simulink model "DFIG"  (Simulink 7.8)
settings: Solver=ode45  StartTime=0.0  StopTime=10.0  RelTol=1e-3
values from neighbouring files (symbols this model uses):
  ps_simStepTime = 5e-6    (= 5e-06)    [plotSimOutput.m]
undefined symbols (not defined in the file or in its folder): D1, Delta, flt_fin_time, flt_start_time, pm_enable_fault, pm_enable_swell, pm_f, pm_fault_type, pm_faultL_H, pm_faultLength, pm_faultR_Ohm, pm_faultStart, pm_gridL_H, pm_gridR_Ohm, pm_initial_angle, pm_multiFault1_end, pm_multiFault1_start, pm_multiFault1L_H, pm_multiFault1R_Ohm, pm_multiFault2_end, pm_multiFault2_start, pm_multiFault2L_H, pm_multiFault2R_Ohm, pm_multiFault3_end, pm_multiFault3_start, pm_multiFault3L_H, pm_multiFault3R_Ohm, pm_multiFault4_end, pm_multiFault4_start, pm_multiFault4L_H, pm_multiFault4R_Ohm, pm_swellaangle_1, pm_swellaangle_2, pm_swellaangle_3, pm_swellbangle_1, pm_swellbangle_2, pm_swellbangle_3, pm_swellcangle_1, pm_swellcangle_2, pm_swellcangle_3, pm_swellEnd, pm_swellPh1_1, pm_swellPh1_2, pm_swellPh1_3, pm_swellPh2_1, pm_swellPh2_2, pm_swellPh2_3, pm_swellPh3_1, pm_swellPh3_2, pm_swellPh3_3, pm_swellStart1, pm_swellStart2, pm_swellStart3, pm_Vg_pp, pm_WTtrafo_L_pu, pm_WTtrafo_Pn_VA, pm_WTtrafo_R_pu, pm_WTtrafo_V2phph_Vrms
libraries: powerlib x39, simulink x4
settings Model: Creator=CNFELUO1  LastModifiedBy=CNFELUO1

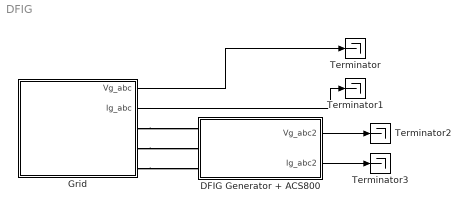
== system DFIG ==
  DFIG Generator + ACS800 : Subsystem
  Grid : Subsystem
  Terminator{,1..3} (4 alike) : Terminator
  wires:
  Grid/1(Vg_abc) -> Terminator/1
  Grid/2(Ig_abc) -> Terminator1/1
  DFIG Generator + ACS800/1(Vg_abc2) -> Terminator2/1
  DFIG Generator + ACS800/2(Ig_abc2) -> Terminator3/1
  connections:
  Grid/RConn3 -- DFIG Generator + ACS800/LConn3
  Grid/RConn2 -- DFIG Generator + ACS800/LConn2
  Grid/RConn1 -- DFIG Generator + ACS800/LConn1

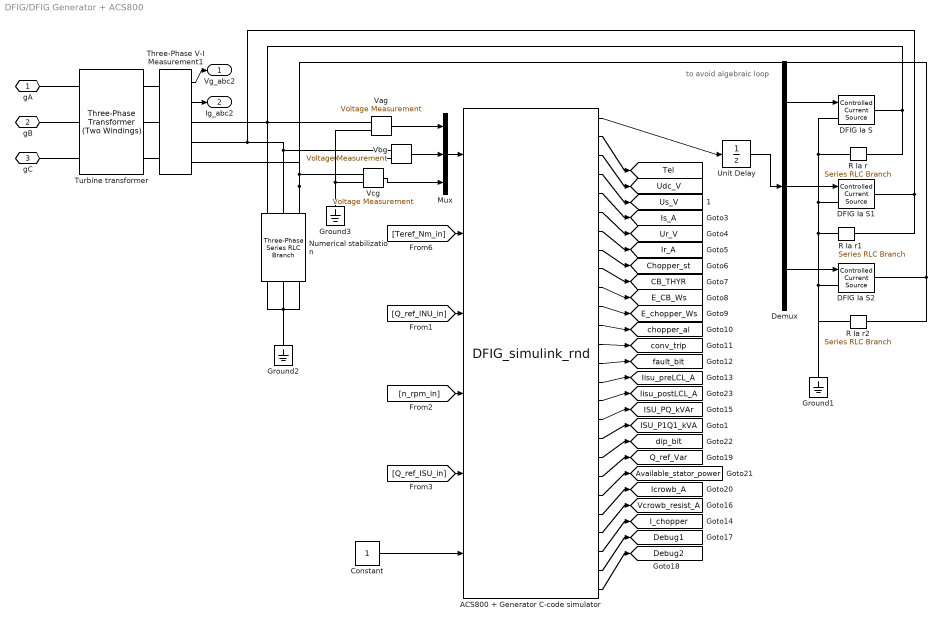
== system DFIG/DFIG Generator + ACS800 ==
  note: to avoid algebraic loop
  ACS800 + Generator C-code simulator : S-Function  FunctionName=DFIG_simulink_rnd  EnableBusSupport=off
      mask Display:
      | port_label('output',1,'Ig_A')
      | port_label('output',2,'Tel')
      | port_label('output',3,'Udc_V')
      | port_label('output',4,'Us_V')
      | port_label('output',5,'Is_A')
      | port_label('output',6,'Ur_V')
      | port_label('output',7,'Ir_A')
      | port_label('output',8,'chopper_st')
      | port_label('output',9,'CB_THYR')
      | port_label('output',10,'E_CB_Ws')
      | port_label('output',11,'E_chopper_Ws')
      | port_label('output',12,'chopper_al')
      | port_label('output',13,'conv_trip')
      | port_label('output',14,'fault_bit')
      | port_label('output',15,'Iisu_preLCL_A')
      | port_label('output',16,'Iisu_postLCL_A')
      | port_label('output',17,'ISU_PQ_kVA')
      | port_label('output',18,'ISU_P1Q1_kVA')
      | port_label('output',19,'dip_bit')
      | port_label('output',20,'Q_ref_VAr')
      | port_label('output',21,'Stator P lim')
      | port_label('output',22,'Icrowb_A')
      | port_label('output',23,'Vcrowb_resist_A')
      | port_label('output',24,'I_chopper')
      | port_label('output',25,'Debug1')
      | port_label('output',26,'Debug2')
      | 
      | port_label('input',1,'Vg_V')
      | port_label('input',2,'Teref_Nm_in')
      | port_label('input',3,'Q_ref_INU_in')
      | port_label('input',4,'n_rpm_in')
      | port_label('input',5,'Q_ref_ISU_in')
      | port_label('input',6,'Enable')
  Constant : Constant
  DFIG Ia S : powerlib/Electrical Sources/Controlled Current Source  Initialize=off  Source_Type=AC  Amplitude=0  Phase=0  Frequency=0  Measurements=None
  DFIG Ia S1 : powerlib/Electrical Sources/Controlled Current Source  Initialize=off  Source_Type=AC  Amplitude=0  Phase=0  Frequency=0  Measurements=None
  DFIG Ia S2 : powerlib/Electrical Sources/Controlled Current Source  Initialize=off  Source_Type=AC  Amplitude=0  Phase=0  Frequency=0  Measurements=None
  Demux : Demux  Outputs=3
  Ground1 : powerlib/Elements/Ground  LConnTagsString=a
  Ground2 : powerlib/Elements/Ground  LConnTagsString=a
  Ground3 : powerlib/Elements/Ground  LConnTagsString=a
  Mux : Mux  Inputs=3
  Numerical stabilization : powerlib/Elements/Three-Phase Series RLC Branch  LConnTagsString=A|B|C  RConnTagsString=A|B|C  BranchType=RC  Resistance=1  Inductance=1e-3  Capacitance=30e-6  Measurements=None
  R Ia r : powerlib/Elements/Series RLC Branch  LConnTagsString=__new0  RConnTagsString=__new0  BranchType=R  Resistance=10e6  Inductance=1e-3  SetiL0=off  InitialCurrent=0  Capacitance=1e-6  Setx0=off  InitialVoltage=0  Measurements=None
  R Ia r1 : powerlib/Elements/Series RLC Branch  LConnTagsString=__new0  RConnTagsString=__new0  BranchType=R  Resistance=10e6  Inductance=1e-3  SetiL0=off  InitialCurrent=0  Capacitance=1e-6  Setx0=off  InitialVoltage=0  Measurements=None
  R Ia r2 : powerlib/Elements/Series RLC Branch  LConnTagsString=__new0  RConnTagsString=__new0  BranchType=R  Resistance=10e6  Inductance=1e-3  SetiL0=off  InitialCurrent=0  Capacitance=1e-6  Setx0=off  InitialVoltage=0  Measurements=None
  Three-Phase V-I Measurement1 : powerlib/Measurements/Three-Phase V-I Measurement  VoltageMeasurement=phase-to-ground  SetLabelV=off  LabelV=Vabc  Vpu=off  VpuLL=off  CurrentMeasurement=yes  SetLabelI=off  LabelI=Iabc  Ipu=off  Pbase=100e6  Vbase=500e3  OutputType=Complex  PhasorSimulation=off  PSBequivalent=0
  Turbine transformer : powerlib/Elements/Three-Phase Transformer (Two Windings)  Winding1Connection=Delta (D1)  UNITS=pu  NominalPower=[ pm_WTtrafo_Pn_VA , pm_f ]  Winding1=[pm_Vg_pp , 0.5*pm_WTtrafo_R_pu , 0.5*pm_WTtrafo_L_pu ]  Winding2Connection=Yg  Winding2=[pm_WTtrafo_V2phph_Vrms , 0.5*pm_WTtrafo_R_pu , 0.5*pm_WTtrafo_L_pu ]  SetSaturation=off  Rm=500  Lm=500  Saturation=[ 0,0 ; 0.0024,1.2 ; 1.0,1.52 ]  Hysteresis=off  DataFile='hysteresis'  SetInitialFlux=off  InitialFluxes=[ 0.8 , -0.8 , 0.7 ]  Measurements=None  MoreParameters=off  BreakLoop=off  DataType=off  TransfoNumber=1
  Unit Delay : UnitDelay  SampleTime=-1
  Vag : powerlib/Measurements/Voltage Measurement  PhasorSimulation=off  OutputType=Complex  PSBequivalent=0
  Vbg : powerlib/Measurements/Voltage Measurement  PhasorSimulation=off  OutputType=Complex  PSBequivalent=0
  Vcg : powerlib/Measurements/Voltage Measurement  PhasorSimulation=off  OutputType=Complex  PSBequivalent=0
  gA : PMIOPort  Port=1  Side=Left
  gB : PMIOPort  Port=2  Side=Left
  gC : PMIOPort  Port=3  Side=Left
  Vg_abc2 : Outport
  Ig_abc2 : Outport  Port=2
  tag scope: Available_stator_power=global, CB_THYR=global, Chopper_st=global, Debug1=global, Debug2=global, E_CB_Ws=global, E_chopper_Ws=global, ISU_P1Q1_kVA=global, ISU_PQ_kVAr=global, I_chopper=global, Icrowb_A=global, Iisu_postLCL_A=global, Iisu_preLCL_A=global, Ir_A=global, Is_A=global, Q_ref_Var=global, Tel=global, Udc_V=global, Ur_V=global, Us_V=global, Vcrowb_resist_A=global, chopper_al=global, conv_trip=global, dip_bit=global, fault_bit=global
  wires:
  ACS800 + Generator C-code simulator/15 -> [Iisu_preLCL_A]
  ACS800 + Generator C-code simulator/14 -> [fault_bit]
  ACS800 + Generator C-code simulator/13 -> [conv_trip]
  ACS800 + Generator C-code simulator/12 -> [chopper_al]
  ACS800 + Generator C-code simulator/11 -> [E_chopper_Ws]
  ACS800 + Generator C-code simulator/10 -> [E_CB_Ws]
  ACS800 + Generator C-code simulator/9 -> [CB_THYR]
  ACS800 + Generator C-code simulator/8 -> [Chopper_st]
  ACS800 + Generator C-code simulator/7 -> [Ir_A]
  ACS800 + Generator C-code simulator/6 -> [Ur_V]
  ACS800 + Generator C-code simulator/5 -> [Is_A]
  ACS800 + Generator C-code simulator/4 -> [Us_V]
  ACS800 + Generator C-code simulator/3 -> [Udc_V]
  ACS800 + Generator C-code simulator/2 -> [Tel]
  Demux/1 -> DFIG Ia S/1
  ACS800 + Generator C-code simulator/1 -> Unit Delay/1
  Mux/1 -> ACS800 + Generator C-code simulator/1
  Demux/2 -> DFIG Ia S1/1
  Demux/3 -> DFIG Ia S2/1
  Unit Delay/1 -> Demux/1
  [Teref_Nm_in] -> ACS800 + Generator C-code simulator/2
  [Q_ref_INU_in] -> ACS800 + Generator C-code simulator/3
  [n_rpm_in] -> ACS800 + Generator C-code simulator/4
  [Q_ref_ISU_in] -> ACS800 + Generator C-code simulator/5
  Vcg/1 -> Mux/3
  Vbg/1 -> Mux/2
  Vag/1 -> Mux/1
  Constant/1 -> ACS800 + Generator C-code simulator/6
  ACS800 + Generator C-code simulator/16 -> [Iisu_postLCL_A]
  ACS800 + Generator C-code simulator/17 -> [ISU_PQ_kVAr]
  ACS800 + Generator C-code simulator/18 -> [ISU_P1Q1_kVA]
  ACS800 + Generator C-code simulator/19 -> [dip_bit]
  ACS800 + Generator C-code simulator/20 -> [Q_ref_Var]
  ACS800 + Generator C-code simulator/21 -> [Available_stator_power]
  ACS800 + Generator C-code simulator/22 -> [Icrowb_A]
  ACS800 + Generator C-code simulator/23 -> [Vcrowb_resist_A]
  ACS800 + Generator C-code simulator/24 -> [I_chopper]
  ACS800 + Generator C-code simulator/25 -> [Debug1]
  ACS800 + Generator C-code simulator/26 -> [Debug2]
  Three-Phase V-I Measurement1/1 -> Vg_abc2/1
  Three-Phase V-I Measurement1/2 -> Ig_abc2/1
  connections:
  Vag/LConn1 -- R Ia r/RConn1 -- DFIG Ia S/RConn1 -- Numerical stabilization/LConn1 -- Three-Phase V-I Measurement1/RConn1
  DFIG Ia S2/RConn1 -- R Ia r2/RConn1 -- Numerical stabilization/LConn3 -- Vcg/LConn1 -- Three-Phase V-I Measurement1/RConn3
  R Ia r1/LConn1 -- R Ia r2/LConn1 -- Ground1/LConn1 -- DFIG Ia S2/LConn1 -- DFIG Ia S1/LConn1 -- DFIG Ia S/LConn1 -- R Ia r/LConn1
  Ground2/LConn1 -- Numerical stabilization/RConn2 -- Numerical stabilization/RConn3 -- Numerical stabilization/RConn1
  Vag/LConn2 -- Vbg/LConn2 -- Ground3/LConn1 -- Vcg/LConn2
  gC/RConn1 -- Turbine transformer/LConn3
  gB/RConn1 -- Turbine transformer/LConn2
  gA/RConn1 -- Turbine transformer/LConn1
  Turbine transformer/RConn1 -- Three-Phase V-I Measurement1/LConn1
  Turbine transformer/RConn2 -- Three-Phase V-I Measurement1/LConn2
  Turbine transformer/RConn3 -- Three-Phase V-I Measurement1/LConn3
  Numerical stabilization/LConn2 -- Vbg/LConn1 -- Three-Phase V-I Measurement1/RConn2 -- R Ia r1/RConn1 -- DFIG Ia S1/RConn1

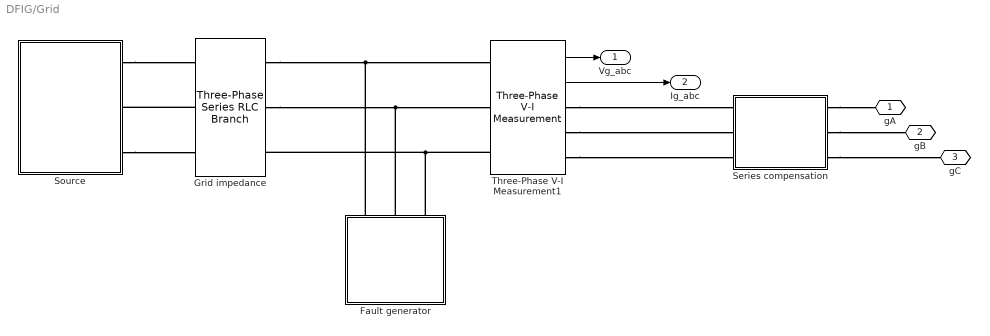
== system DFIG/Grid ==
  Fault generator : Subsystem
  Grid impedance : powerlib/Elements/Three-Phase Series RLC Branch  LConnTagsString=A|B|C  RConnTagsString=A|B|C  BranchType=RL  Resistance=pm_gridR_Ohm  Inductance=pm_gridL_H  Capacitance=[]  Measurements=None
  Series compensation : Subsystem  mask{t_on=3, c=5e-4}
      mask prompts: t_on "Compensation switch on time (s)"; c "Series capacitance (F)"
  Source : Subsystem
  Three-Phase V-I Measurement1 : powerlib/Measurements/Three-Phase V-I Measurement  VoltageMeasurement=phase-to-ground  SetLabelV=off  LabelV=Vabc  Vpu=off  VpuLL=off  CurrentMeasurement=yes  SetLabelI=off  LabelI=Iabc  Ipu=off  Pbase=100e6  Vbase=500e3  OutputType=Complex  PhasorSimulation=off  PSBequivalent=0
  gA : PMIOPort  Port=1  Side=Right
  gB : PMIOPort  Port=2  Side=Right
  gC : PMIOPort  Port=3  Side=Right
  Vg_abc : Outport
  Ig_abc : Outport  Port=2
  wires:
  Three-Phase V-I Measurement1/2 -> Ig_abc/1
  Three-Phase V-I Measurement1/1 -> Vg_abc/1
  connections:
  Three-Phase V-I Measurement1/LConn3 -- Grid impedance/RConn3 -- Fault generator/RConn3
  Grid impedance/RConn2 -- Three-Phase V-I Measurement1/LConn2 -- Fault generator/RConn2
  Grid impedance/RConn1 -- Three-Phase V-I Measurement1/LConn1 -- Fault generator/RConn1
  Source/RConn1 -- Grid impedance/LConn1
  Grid impedance/LConn2 -- Source/RConn2
  Source/RConn3 -- Grid impedance/LConn3
  Three-Phase V-I Measurement1/RConn1 -- Series compensation/RConn1
  Three-Phase V-I Measurement1/RConn2 -- Series compensation/RConn2
  Three-Phase V-I Measurement1/RConn3 -- Series compensation/RConn3
  Series compensation/LConn1 -- gA/RConn1
  Series compensation/LConn2 -- gB/RConn1
  Series compensation/LConn3 -- gC/RConn1

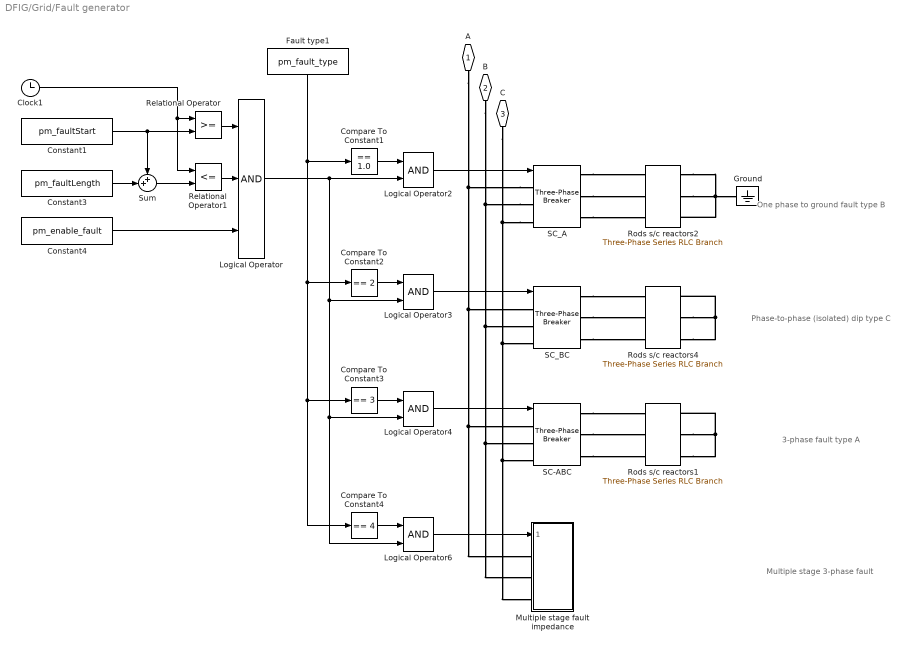
== system DFIG/Grid/Fault generator ==
  note: Multiple stage 3-phase fault
  note: One phase to ground fault
      | type B
  note: 3-phase fault
      | type A
  note: Phase-to-phase (isolated) dip
      | type C
  Clock1 : Clock
  Compare To Constant1 : simulink/Logic and Bit Operations/Compare To Constant  relop===  const=1.0  OutDataTypeStr=uint8
  Compare To Constant2 : simulink/Logic and Bit Operations/Compare To Constant  relop===  const=2  OutDataTypeStr=uint8
  Compare To Constant3 : simulink/Logic and Bit Operations/Compare To Constant  relop===  const=3  OutDataTypeStr=uint8
  Compare To Constant4 : simulink/Logic and Bit Operations/Compare To Constant  relop===  const=4  OutDataTypeStr=uint8
  Constant1 : Constant  Value=pm_faultStart
  Constant3 : Constant  Value=pm_faultLength
  Constant4 : Constant  Value=pm_enable_fault
  Fault type1 : Constant  Value=pm_fault_type
  Ground : powerlib/Elements/Ground  LConnTagsString=a
  Logical Operator : Logic  Inputs=3  AllPortsSameDT=off  OutDataTypeStr=boolean
  Logical Operator{2..4,6} (4 alike) : Logic  AllPortsSameDT=off  OutDataTypeStr=boolean
  Multiple stage fault impedance : Subsystem
  Relational Operator : RelationalOperator  OutDataTypeStr=boolean
  Relational Operator1 : RelationalOperator  Operator=<=  OutDataTypeStr=boolean
  Rods s/c reactors1 : powerlib/Elements/Three-Phase Series RLC Branch  LConnTagsString=A|B|C  RConnTagsString=A|B|C  BranchType=RL  Resistance=pm_faultR_Ohm  Inductance=pm_faultL_H  Capacitance=[]  Measurements=None
  Rods s/c reactors2 : powerlib/Elements/Three-Phase Series RLC Branch  LConnTagsString=A|B|C  RConnTagsString=A|B|C  BranchType=RL  Resistance=pm_faultR_Ohm  Inductance=pm_faultL_H  Capacitance=[]  Measurements=None
  Rods s/c reactors4 : powerlib/Elements/Three-Phase Series RLC Branch  LConnTagsString=A|B|C  RConnTagsString=A|B|C  BranchType=RL  Resistance=pm_faultR_Ohm  Inductance=pm_faultL_H  Capacitance=[]  Measurements=None
  SC-ABC : powerlib/Elements/Three-Phase Breaker  InitialState=open  SwitchA=on  SwitchB=on  SwitchC=on  SwitchTimes="[flt_start_time  flt_fin_time]"  External=on  BreakerResistance=1e-6  SnubberResistance=10000000  SnubberCapacitance=inf  Measurements=None
      settings: AttributesFormatString=\n
  SC_A : powerlib/Elements/Three-Phase Breaker  InitialState=open  SwitchA=on  SwitchB=off  SwitchC=off  SwitchTimes="[flt_start_time  flt_fin_time]"  External=on  BreakerResistance=1e-6  SnubberResistance=10000000  SnubberCapacitance=inf  Measurements=None
      settings: AttributesFormatString=\n
  SC_BC : powerlib/Elements/Three-Phase Breaker  InitialState=open  SwitchA=off  SwitchB=on  SwitchC=on  SwitchTimes="[flt_start_time  flt_fin_time]"  External=on  BreakerResistance=1e-6  SnubberResistance=10000000  SnubberCapacitance=inf  Measurements=None
      settings: AttributesFormatString=\n
  Sum : Sum  Inputs=++|
  A : PMIOPort  Port=1  Side=Right
  B : PMIOPort  Port=2  Side=Right
  C : PMIOPort  Port=3  Side=Right
  wires:
  Clock1/1 -> Relational Operator/1, Relational Operator1/1
  Logical Operator/1 -> Logical Operator6/2, Logical Operator4/2, Logical Operator3/2, Logical Operator2/2
  Constant4/1 -> Logical Operator/3
  Relational Operator1/1 -> Logical Operator/2
  Relational Operator/1 -> Logical Operator/1
  Sum/1 -> Relational Operator1/2
  Constant1/1 -> Relational Operator/2, Sum/1
  Constant3/1 -> Sum/2
  Logical Operator6/1 -> Multiple stage fault impedance/1(Enabled)
  Logical Operator4/1 -> SC-ABC/1
  Logical Operator3/1 -> SC_BC/1
  Logical Operator2/1 -> SC_A/1
  Compare To Constant4/1 -> Logical Operator6/1
  Compare To Constant3/1 -> Logical Operator4/1
  Compare To Constant2/1 -> Logical Operator3/1
  Fault type1/1 -> Compare To Constant4/1, Compare To Constant3/1, Compare To Constant2/1, Compare To Constant1/1
  Compare To Constant1/1 -> Logical Operator2/1
  connections:
  SC_A/LConn1 -- SC_BC/LConn1 -- SC-ABC/LConn1 -- Multiple stage fault impedance/LConn1 -- A/RConn1
  SC_A/LConn2 -- SC_BC/LConn2 -- SC-ABC/LConn2 -- Multiple stage fault impedance/LConn2 -- B/RConn1
  SC_A/LConn3 -- SC_BC/LConn3 -- SC-ABC/LConn3 -- Multiple stage fault impedance/LConn3 -- C/RConn1
  SC_A/RConn1 -- Rods s/c reactors2/LConn1
  SC_A/RConn2 -- Rods s/c reactors2/LConn2
  SC_A/RConn3 -- Rods s/c reactors2/LConn3
  Rods s/c reactors2/RConn2 -- Rods s/c reactors2/RConn3 -- Rods s/c reactors2/RConn1 -- Ground/LConn1
  SC-ABC/RConn1 -- Rods s/c reactors1/LConn1
  SC-ABC/RConn2 -- Rods s/c reactors1/LConn2
  SC-ABC/RConn3 -- Rods s/c reactors1/LConn3
  Rods s/c reactors1/RConn3 -- Rods s/c reactors1/RConn1 -- Rods s/c reactors1/RConn2
  Rods s/c reactors4/RConn2 -- Rods s/c reactors4/RConn1 -- Rods s/c reactors4/RConn3
  SC_BC/RConn1 -- Rods s/c reactors4/LConn1
  SC_BC/RConn2 -- Rods s/c reactors4/LConn2
  SC_BC/RConn3 -- Rods s/c reactors4/LConn3

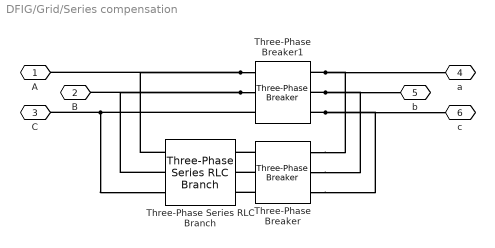
== system DFIG/Grid/Series compensation ==
  Three-Phase Series RLC Branch : powerlib/Elements/Three-Phase Series RLC Branch  LConnTagsString=A|B|C  RConnTagsString=A|B|C  BranchType=C  Resistance=1  Inductance=1e-3  Capacitance=c  Measurements=None
  Three-Phase Breaker : powerlib/Elements/Three-Phase Breaker  InitialState=open  SwitchA=on  SwitchB=on  SwitchC=on  SwitchTimes=[t_on]  External=off  BreakerResistance=0.001  SnubberResistance=1e6  SnubberCapacitance=inf  Measurements=None
  Three-Phase Breaker1 : powerlib/Elements/Three-Phase Breaker  InitialState=closed  SwitchA=on  SwitchB=on  SwitchC=on  SwitchTimes=[t_on]  External=off  BreakerResistance=0.001  SnubberResistance=1e6  SnubberCapacitance=inf  Measurements=None
  A : PMIOPort  Port=1  Side=Right
  B : PMIOPort  Port=2  Side=Right
  C : PMIOPort  Port=3  Side=Right
  a : PMIOPort  Port=4  Side=Left
  b : PMIOPort  Port=5  Side=Left
  c : PMIOPort  Port=6  Side=Left
  connections:
  Three-Phase Breaker1/RConn3 -- c/RConn1 -- Three-Phase Breaker/RConn3
  Three-Phase Breaker1/RConn2 -- b/RConn1 -- Three-Phase Breaker/RConn2
  Three-Phase Breaker1/RConn1 -- a/RConn1 -- Three-Phase Breaker/RConn1
  Three-Phase Breaker/LConn3 -- Three-Phase Series RLC Branch/RConn3
  Three-Phase Breaker/LConn2 -- Three-Phase Series RLC Branch/RConn2
  Three-Phase Breaker/LConn1 -- Three-Phase Series RLC Branch/RConn1
  Three-Phase Breaker1/LConn3 -- C/RConn1 -- Three-Phase Series RLC Branch/LConn3
  Three-Phase Breaker1/LConn2 -- B/RConn1 -- Three-Phase Series RLC Branch/LConn2
  Three-Phase Breaker1/LConn1 -- A/RConn1 -- Three-Phase Series RLC Branch/LConn1

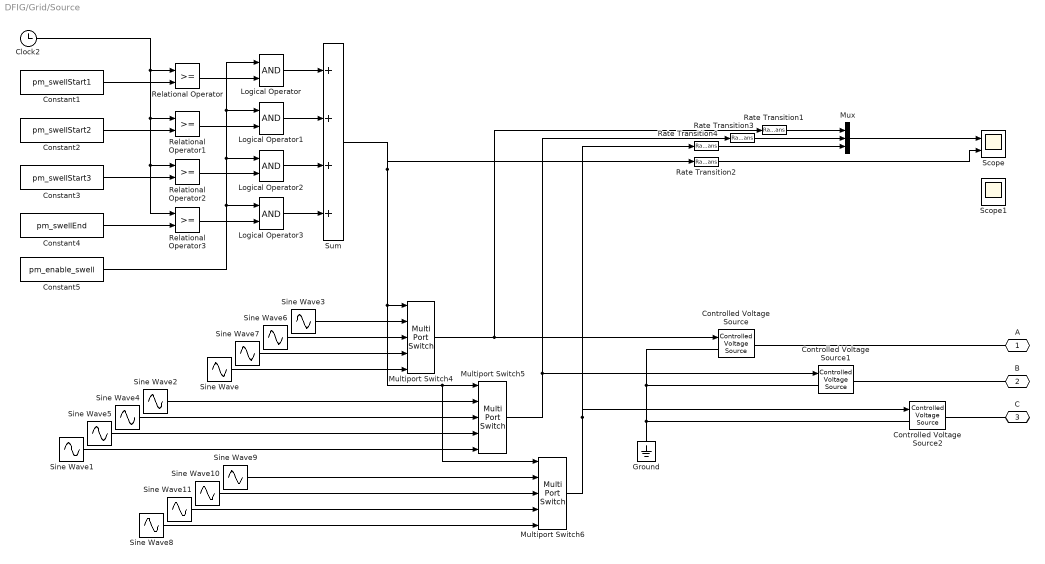
== system DFIG/Grid/Source ==
  Clock2 : Clock
  Constant1 : Constant  Value=pm_swellStart1
  Constant2 : Constant  Value=pm_swellStart2
  Constant3 : Constant  Value=pm_swellStart3
  Constant4 : Constant  Value=pm_swellEnd
  Constant5 : Constant  Value=pm_enable_swell
  Controlled Voltage Source : powerlib/Electrical Sources/Controlled Voltage Source  Initialize=on  Source_Type=AC  Amplitude=0  Phase=0  Frequency=0  Measurements=None
  Controlled Voltage Source1 : powerlib/Electrical Sources/Controlled Voltage Source  Initialize=on  Source_Type=AC  Amplitude=0  Phase=0  Frequency=0  Measurements=None
  Controlled Voltage Source2 : powerlib/Electrical Sources/Controlled Voltage Source  Initialize=on  Source_Type=AC  Amplitude=0  Phase=0  Frequency=0  Measurements=None
  Ground : powerlib/Elements/Ground  LConnTagsString=a
  Logical Operator{,1..3} (4 alike) : Logic  AllPortsSameDT=off  OutDataTypeStr=boolean
  Multiport Switch4 : MultiPortSwitch  Inputs=4  zeroidx=off
  Multiport Switch5 : MultiPortSwitch  Inputs=4  zeroidx=off
  Multiport Switch6 : MultiPortSwitch  Inputs=4  zeroidx=off
  Mux : Mux  Inputs=3
  Rate Transition{1..4} (4 alike) : RateTransition  OutPortSampleTime=500e-6
  Relational Operator{,1..3} (4 alike) : RelationalOperator  OutDataTypeStr=boolean
  Scope : Scope  NumInputPorts=2
      settings: YMin=-30000~-5  YMax=30000~5
  Scope1 : Scope  NumInputPorts=2
      settings: YMin=-30000~-5  YMax=30000~5
  Sine Wave : Sin  Amplitude=pm_Vg_pp*sqrt(2)./sqrt(3)  Frequency=pm_f*2*pi  Phase=pm_initial_angle.*pi./180  SampleTime=ps_simStepTime  VectorParams1D=off
  Sine Wave1 : Sin  Amplitude=pm_Vg_pp*sqrt(2)./sqrt(3)  Frequency=pm_f*2*pi  Phase=pm_initial_angle.*pi./180-2*pi/3  SampleTime=ps_simStepTime  VectorParams1D=off
  Sine Wave10 : Sin  Amplitude=pm_Vg_pp*sqrt(2)./sqrt(3)*pm_swellPh3_2  Frequency=pm_f*2*pi  Phase=pm_initial_angle.*pi./180 + pm_swellcangle_2  SampleTime=ps_simStepTime  VectorParams1D=off
  Sine Wave11 : Sin  Amplitude=pm_Vg_pp*sqrt(2)./sqrt(3)*pm_swellPh3_3  Frequency=pm_f*2*pi  Phase=pm_initial_angle.*pi./180+pm_swellcangle_3  SampleTime=ps_simStepTime  VectorParams1D=off
  Sine Wave2 : Sin  Amplitude=pm_Vg_pp*sqrt(2)./sqrt(3)*pm_swellPh2_1  Frequency=pm_f*2*pi  Phase=pm_initial_angle.*pi./180+pm_swellbangle_1  SampleTime=ps_simStepTime  VectorParams1D=off
  Sine Wave3 : Sin  Amplitude=pm_Vg_pp*sqrt(2)./sqrt(3)*pm_swellPh1_1  Frequency=pm_f*2*pi  Phase=pm_initial_angle.*pi./180+pm_swellaangle_1  SampleTime=ps_simStepTime  VectorParams1D=off
  Sine Wave4 : Sin  Amplitude=pm_Vg_pp*sqrt(2)./sqrt(3)*pm_swellPh2_2  Frequency=pm_f*2*pi  Phase=pm_initial_angle.*pi./180+pm_swellbangle_2  SampleTime=ps_simStepTime  VectorParams1D=off
  Sine Wave5 : Sin  Amplitude=pm_Vg_pp*sqrt(2)./sqrt(3)*pm_swellPh2_3  Frequency=pm_f*2*pi  Phase=pm_initial_angle.*pi./180+pm_swellbangle_3  SampleTime=ps_simStepTime  VectorParams1D=off
  Sine Wave6 : Sin  Amplitude=pm_Vg_pp*sqrt(2)./sqrt(3)*pm_swellPh1_2  Frequency=pm_f*2*pi  Phase=pm_initial_angle.*pi./180+pm_swellaangle_2  SampleTime=ps_simStepTime  VectorParams1D=off
  Sine Wave7 : Sin  Amplitude=pm_Vg_pp*sqrt(2)./sqrt(3)*pm_swellPh1_3  Frequency=pm_f*2*pi  Phase=pm_initial_angle.*pi./180+pm_swellaangle_3  SampleTime=ps_simStepTime  VectorParams1D=off
  Sine Wave8 : Sin  Amplitude=pm_Vg_pp*sqrt(2)./sqrt(3)  Frequency=pm_f*2*pi  Phase=pm_initial_angle.*pi./180 - 4*pi/3  SampleTime=ps_simStepTime  VectorParams1D=off
  Sine Wave9 : Sin  Amplitude=pm_Vg_pp*sqrt(2)./sqrt(3)*pm_swellPh3_1  Frequency=pm_f*2*pi  Phase=pm_initial_angle.*pi./180+pm_swellcangle_1  SampleTime=ps_simStepTime  VectorParams1D=off
  Sum : Sum  Inputs=++++
  A : PMIOPort  Port=1  Side=Right
  B : PMIOPort  Port=2  Side=Right
  C : PMIOPort  Port=3  Side=Right
  wires:
  Constant1/1 -> Relational Operator/2
  Clock2/1 -> Relational Operator/1, Relational Operator1/1, Relational Operator2/1, Relational Operator3/1
  Constant2/1 -> Relational Operator1/2
  Constant3/1 -> Relational Operator2/2
  Constant4/1 -> Relational Operator3/2
  Multiport Switch5/1 -> Controlled Voltage Source1/1, Rate Transition3/1
  Multiport Switch6/1 -> Controlled Voltage Source2/1, Rate Transition4/1
  Sine Wave3/1 -> Multiport Switch4/2
  Sine Wave6/1 -> Multiport Switch4/3
  Sine Wave7/1 -> Multiport Switch4/4
  Sine Wave2/1 -> Multiport Switch5/2
  Sine Wave4/1 -> Multiport Switch5/3
  Sine Wave5/1 -> Multiport Switch5/4
  Sine Wave1/1 -> Multiport Switch5/5
  Sine Wave9/1 -> Multiport Switch6/2
  Sine Wave10/1 -> Multiport Switch6/3
  Sine Wave11/1 -> Multiport Switch6/4
  Sine Wave8/1 -> Multiport Switch6/5
  Sine Wave/1 -> Multiport Switch4/5
  Sum/1 -> Multiport Switch4/1, Multiport Switch5/1, Multiport Switch6/1, Rate Transition2/1
  Relational Operator/1 -> Logical Operator/2
  Relational Operator1/1 -> Logical Operator1/2
  Relational Operator2/1 -> Logical Operator2/2
  Relational Operator3/1 -> Logical Operator3/2
  Constant5/1 -> Logical Operator3/1, Logical Operator2/1, Logical Operator1/1, Logical Operator/1
  Logical Operator/1 -> Sum/1
  Logical Operator2/1 -> Sum/3
  Logical Operator1/1 -> Sum/2
  Logical Operator3/1 -> Sum/4
  Multiport Switch4/1 -> Controlled Voltage Source/1, Rate Transition1/1
  Mux/1 -> Scope/1
  Rate Transition1/1 -> Mux/1
  Rate Transition3/1 -> Mux/2
  Rate Transition4/1 -> Mux/3
  Rate Transition2/1 -> Scope/2
  connections:
  A/RConn1 -- Controlled Voltage Source/RConn1
  B/RConn1 -- Controlled Voltage Source1/RConn1
  C/RConn1 -- Controlled Voltage Source2/RConn1
  Ground/LConn1 -- Controlled Voltage Source2/LConn1 -- Controlled Voltage Source/LConn1 -- Controlled Voltage Source1/LConn1

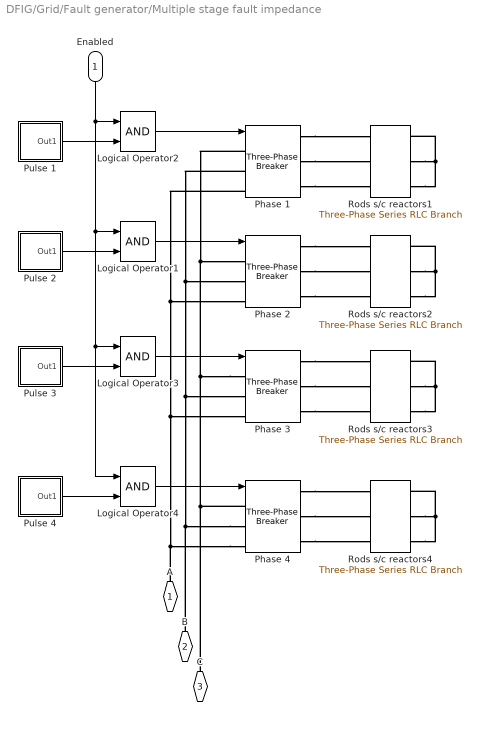
== system DFIG/Grid/Fault generator/Multiple stage fault impedance ==
  Enabled : Inport
  Logical Operator{1..4} (4 alike) : Logic  AllPortsSameDT=off  OutDataTypeStr=boolean
  Phase {1..4} (4 alike) : powerlib/Elements/Three-Phase Breaker  InitialState=open  SwitchA=on  SwitchB=on  SwitchC=on  SwitchTimes="[flt_start_time  flt_fin_time]"  External=on  BreakerResistance=1e-6  SnubberResistance=10000000  SnubberCapacitance=inf  Measurements=None
      settings: AttributesFormatString=\n
  Pulse 1 : Subsystem  mask{pulseStart=pm_multiFault1_start, pulseEnd=pm_multiFault1_end}
      mask prompts: pulseStart "Pulse start time (s)"; pulseEnd "Pulse end time (s)"
      mask Display: plot([10 20 20 30 30 40],[0 0 10 10 0 0])
  Pulse 2 : Subsystem  mask{pulseStart=pm_multiFault2_start, pulseEnd=pm_multiFault2_end}
      mask prompts: pulseStart "Pulse start time (s)"; pulseEnd "Pulse end time (s)"
      mask Display: plot([10 20 20 30 30 40],[0 0 10 10 0 0])
  Pulse 3 : Subsystem  mask{pulseStart=pm_multiFault3_start, pulseEnd=pm_multiFault3_end}
      mask prompts: pulseStart "Pulse start time (s)"; pulseEnd "Pulse end time (s)"
      mask Display: plot([10 20 20 30 30 40],[0 0 10 10 0 0])
  Pulse 4 : Subsystem  mask{pulseStart=pm_multiFault4_start, pulseEnd=pm_multiFault4_end}
      mask prompts: pulseStart "Pulse start time (s)"; pulseEnd "Pulse end time (s)"
      mask Display: plot([10 20 20 30 30 40],[0 0 10 10 0 0])
  Rods s/c reactors1 : powerlib/Elements/Three-Phase Series RLC Branch  LConnTagsString=A|B|C  RConnTagsString=A|B|C  BranchType=RL  Resistance=pm_multiFault1R_Ohm  Inductance=pm_multiFault1L_H  Capacitance=[]  Measurements=None
  Rods s/c reactors2 : powerlib/Elements/Three-Phase Series RLC Branch  LConnTagsString=A|B|C  RConnTagsString=A|B|C  BranchType=RL  Resistance=pm_multiFault2R_Ohm  Inductance=pm_multiFault2L_H  Capacitance=[]  Measurements=None
  Rods s/c reactors3 : powerlib/Elements/Three-Phase Series RLC Branch  LConnTagsString=A|B|C  RConnTagsString=A|B|C  BranchType=RL  Resistance=pm_multiFault3R_Ohm  Inductance=pm_multiFault3L_H  Capacitance=[]  Measurements=None
  Rods s/c reactors4 : powerlib/Elements/Three-Phase Series RLC Branch  LConnTagsString=A|B|C  RConnTagsString=A|B|C  BranchType=RL  Resistance=pm_multiFault4R_Ohm  Inductance=pm_multiFault4L_H  Capacitance=[]  Measurements=None
  A : PMIOPort  Port=1  Side=Left
  B : PMIOPort  Port=2  Side=Left
  C : PMIOPort  Port=3  Side=Left
  wires:
  Enabled/1 -> Logical Operator4/1, Logical Operator3/1, Logical Operator1/1, Logical Operator2/1
  Pulse 1/1(Out1) -> Logical Operator2/2
  Pulse 2/1(Out1) -> Logical Operator1/2
  Pulse 3/1(Out1) -> Logical Operator3/2
  Pulse 4/1(Out1) -> Logical Operator4/2
  Logical Operator4/1 -> Phase 4/1
  Logical Operator3/1 -> Phase 3/1
  Logical Operator1/1 -> Phase 2/1
  Logical Operator2/1 -> Phase 1/1
  connections:
  Phase 4/RConn3 -- Rods s/c reactors4/LConn3
  Phase 2/RConn3 -- Rods s/c reactors2/LConn3
  Phase 3/RConn2 -- Rods s/c reactors3/LConn2
  Phase 3/RConn3 -- Rods s/c reactors3/LConn3
  Phase 3/RConn1 -- Rods s/c reactors3/LConn1
  Phase 1/RConn3 -- Rods s/c reactors1/LConn3
  Phase 1/RConn2 -- Rods s/c reactors1/LConn2
  Phase 2/RConn1 -- Rods s/c reactors2/LConn1
  Phase 2/RConn2 -- Rods s/c reactors2/LConn2
  Phase 4/RConn2 -- Rods s/c reactors4/LConn2
  Phase 1/RConn1 -- Rods s/c reactors1/LConn1
  Phase 4/RConn1 -- Rods s/c reactors4/LConn1
  Rods s/c reactors4/RConn2 -- Rods s/c reactors4/RConn3 -- Rods s/c reactors4/RConn1
  Rods s/c reactors3/RConn2 -- Rods s/c reactors3/RConn3 -- Rods s/c reactors3/RConn1
  Rods s/c reactors2/RConn2 -- Rods s/c reactors2/RConn3 -- Rods s/c reactors2/RConn1
  Rods s/c reactors1/RConn2 -- Rods s/c reactors1/RConn3 -- Rods s/c reactors1/RConn1
  Phase 4/LConn2 -- Phase 3/LConn2 -- Phase 1/LConn2 -- Phase 2/LConn2 -- B/RConn1
  Phase 4/LConn3 -- Phase 3/LConn3 -- Phase 1/LConn3 -- Phase 2/LConn3 -- A/RConn1
  Phase 3/LConn1 -- Phase 1/LConn1 -- Phase 2/LConn1 -- Phase 4/LConn1 -- C/RConn1

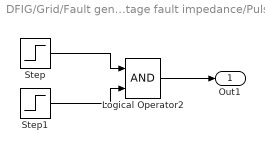
== system DFIG/Grid/Fault generator/Multiple stage fault impedance/Pulse 1 ==
  Logical Operator2 : Logic  AllPortsSameDT=off  OutDataTypeStr=boolean
  Step : Step  Time=pulseStart  SampleTime=0
  Step1 : Step  Time=pulseEnd  Before=1  After=0  SampleTime=0
  Out1 : Outport
  wires:
  Logical Operator2/1 -> Out1/1
  Step1/1 -> Logical Operator2/2
  Step/1 -> Logical Operator2/1

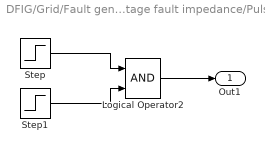
== system DFIG/Grid/Fault generator/Multiple stage fault impedance/Pulse 2 ==
  Logical Operator2 : Logic  AllPortsSameDT=off  OutDataTypeStr=boolean
  Step : Step  Time=pulseStart  SampleTime=0
  Step1 : Step  Time=pulseEnd  Before=1  After=0  SampleTime=0
  Out1 : Outport
  wires:
  Step/1 -> Logical Operator2/1
  Step1/1 -> Logical Operator2/2
  Logical Operator2/1 -> Out1/1

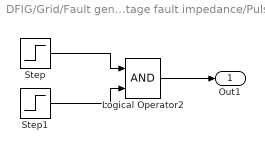
== system DFIG/Grid/Fault generator/Multiple stage fault impedance/Pulse 3 ==
  Logical Operator2 : Logic  AllPortsSameDT=off  OutDataTypeStr=boolean
  Step : Step  Time=pulseStart  SampleTime=0
  Step1 : Step  Time=pulseEnd  Before=1  After=0  SampleTime=0
  Out1 : Outport
  wires:
  Logical Operator2/1 -> Out1/1
  Step1/1 -> Logical Operator2/2
  Step/1 -> Logical Operator2/1

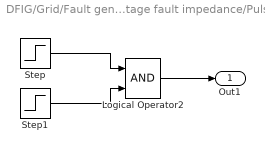
== system DFIG/Grid/Fault generator/Multiple stage fault impedance/Pulse 4 ==
  Logical Operator2 : Logic  AllPortsSameDT=off  OutDataTypeStr=boolean
  Step : Step  Time=pulseStart  SampleTime=0
  Step1 : Step  Time=pulseEnd  Before=1  After=0  SampleTime=0
  Out1 : Outport
  wires:
  Step/1 -> Logical Operator2/1
  Step1/1 -> Logical Operator2/2
  Logical Operator2/1 -> Out1/1
